simulink library "inp"  (Simulink 7.4)
settings: Solver=ode45  StartTime=0.0  StopTime=10.0  RelTol=1e-3
undefined symbols (not defined in the file): AINP_BrkPedalInterp_X_bar, C_TASK_10MS_S, ENUM_SHIFTER_D, ENUM_SHIFTER_N, ENUM_SHIFTER_P, ENUM_SHIFTER_R, KINP_BonnetCloseVehSpdThre_kph, KINP_EDUCoolantTempFilTm_s, KINP_EDUOilPressureFilTm_s, KINP_EDUOilTempFilTm_s, KINP_EDUSynchDisp_mm, KINP_EDUSynchPosnPWMDC_pct_LowerLimit, KINP_EDUSynchPosnPWMDC_pct_ovrdflg, KINP_EDUSynchPosnPWMDC_pct_ovrdval, KINP_EDUSynchPosnPWMDC_pct_UpperLimit, KINP_ShifterPosConfirmD_s, KINP_ShifterPosConfirmN_s, KINP_ShifterPosConfirmP_s, KINP_ShifterPosConfirmR_s, KINP_SingleAccPedalFltRateLim_pct, KINP_TMSpd2VehSpdSigNeg_rpm, KINP_TMSpd2VehSpdSigPos_rpm, KINP_ValidCheck_EDUSynchPosnPWMDC_dec, KINP_ValidCheck_EDUSynchPosnPWMDC_inc, KINP_ValidCheck_EDUSynchPosnPWMDC_lim, KINP_VehSpdSigKeepThres_kph, KPH2MPS, MIN2SEC, MINP_BrkPedalInterp_pct, MPS2KPH, PI, seat_version_control_block_callbacks, TIRE_RADIUS
libraries: inp_lib x166, hcu_lib x4, simulink x1
(part 3 of 9)

== system inp/INP/INP_100MS/Message (100ms) ISC_HSC2_FrP02 ==
  BHAL_IN_100ms : Inport
  BSRV_In_ovrdflgs : Inport  Port=2
  BSRV_In_ovrdvals : Inport  Port=3
  VINP_ISCMsgAlive_flg : Inport  Port=4
  Bus Creator : BusCreator  Inputs=6
  Bus Selector1 : BusSelector  OutputSignals=VSRV_ISGOverTempIn_flg_ovrdflg
  Bus Selector10 : BusSelector  OutputSignals=VHAL_ISGDeratingIn_flg
  Bus Selector12 : BusSelector  OutputSignals=VSRV_DCDCTempIn_C_ovrdflg
  Bus Selector14 : BusSelector  OutputSignals=VSRV_DCDCLVLoadIn_pct_ovrdflg
  Bus Selector16 : BusSelector  OutputSignals=VSRV_DCDCLVLoadIn_pct_ovrdval
  Bus Selector17 : BusSelector  OutputSignals=VHAL_DCDCLVLoadIn_pct
  Bus Selector2 : BusSelector  OutputSignals=VSRV_ISCHSC2FrP02Active_flg_ovrdflg
  Bus Selector3 : BusSelector  OutputSignals=VSRV_ISCHSC2FrP02Active_flg_ovrdval
  Bus Selector4 : BusSelector  OutputSignals=VHAL_DCDCTempValidIn_flg
  Bus Selector43 : BusSelector  OutputSignals=VSRV_DCDCFaultIn_flg_ovrdflg
  Bus Selector44 : BusSelector  OutputSignals=VSRV_DCDCFaultIn_flg_ovrdval
  Bus Selector45 : BusSelector  OutputSignals=VHAL_DCDCFaultIn_flg
  Bus Selector46 : BusSelector  OutputSignals=VSRV_DCDCTempIn_C_ovrdval
  Bus Selector47 : BusSelector  OutputSignals=VHAL_DCDCTempIn_C
  Bus Selector5 : BusSelector  OutputSignals=VSRV_ISGOverTempIn_flg_ovrdval
  Bus Selector6 : BusSelector  OutputSignals=VHAL_DCDCLVLoadValidIn_flg
  Bus Selector7 : BusSelector  OutputSignals=VHAL_ISGOverTempIn_flg
  Bus Selector8 : BusSelector  OutputSignals=VSRV_ISGDeratingIn_flg_ovrdflg
  Bus Selector9 : BusSelector  OutputSignals=VSRV_ISGDeratingIn_flg_ovrdval
  Subsys VINP_DCDCFault_flg : inp_lib/msgactv_ovrd  SystemSampleTime=-1  cal_ovrdflg=KINP_DCDCFault_flg_ovrdflg  cal_ovrdval=KINP_DCDCFault_flg_ovrdval  default=KINP_DCDCFaultDefault_flg
  Subsys VINP_DCDCLVLoad_pct : inp_lib/valid_msgactv_sat_ovrd  SystemSampleTime=-1  cal_ovrdflg=KINP_DCDCLVLoad_pct_ovrdflg  cal_ovrdval=KINP_DCDCLVLoad_pct_ovrdval  lim=KINP_ValidCheck_DCDCLVLoad_lim  inc=KINP_ValidCheck_DCDCLVLoad_inc  dec=KINP_ValidCheck_DCDCLVLoad_dec  default=KINP_DCDCLVLoadDefault_pct  hi=KINP_DCDCLVLoad_pct_Max  lo=KINP_DCDCLVLoad_pct_Min
  Subsys VINP_DCDCTemp_C : inp_lib/valid_msgactv_sat_ovrd  SystemSampleTime=-1  cal_ovrdflg=KINP_DCDCTemp_C_ovrdflg  cal_ovrdval=KINP_DCDCTemp_C_ovrdval  lim=KINP_ValidCheck_DCDCTemp_lim  inc=KINP_ValidCheck_DCDCTemp_inc  dec=KINP_ValidCheck_DCDCTemp_dec  default=KINP_DCDCTempDefault_C  hi=KINP_DCDCTemp_C_Max  lo=KINP_DCDCTemp_C_Min
  Subsys VINP_ISCHSC2FrP02Active_flg : inp_lib/override  SystemSampleTime=-1  cal_ovrdflg=KINP_ISCHSC2FrP02Active_ovrdflg  cal_ovrdval=KINP_ISCHSC2FrP02Active_flg_ovrdval
  Subsys VINP_ISGDerating_flg : inp_lib/msgactv_ovrd  SystemSampleTime=-1  cal_ovrdflg=KINP_ISGDerating_flg_ovrdflg  cal_ovrdval=KINP_ISGDerating_flg_ovrdval  default=KINP_ISGDeratingDefault_flg
  Subsys VINP_ISGOverTemp_flg : inp_lib/msgactv_ovrd  SystemSampleTime=-1  cal_ovrdflg=KINP_ISGOverTemp_flg_ovrdflg  cal_ovrdval=KINP_ISGOverTemp_flg_ovrdval  default=KINP_ISGOverTempDefault_flg
  Terminator{,1..4} (5 alike) : Terminator
  BINP_ISC_HSC2_FrP02 : Outport
  wires:
  [BSRV_In_ovrdvals] -> Bus Selector9/1
  [BSRV_In_ovrdflgs] -> Bus Selector8/1
  [BSRV_In_ovrdvals] -> Bus Selector5/1
  [BSRV_In_ovrdflgs] -> Bus Selector1/1
  [BSRV_In_ovrdvals] -> Bus Selector3/1
  [BSRV_In_ovrdflgs] -> Bus Selector2/1
  [BSRV_In_ovrdvals] -> Bus Selector46/1
  [BSRV_In_ovrdflgs] -> Bus Selector12/1
  [BSRV_In_ovrdvals] -> Bus Selector44/1
  [BSRV_In_ovrdflgs] -> Bus Selector43/1
  BHAL_IN_100ms/1 -> Bus Selector10/1, Bus Selector7/1, Bus Selector47/1, Bus Selector4/1, Bus Selector6/1, Bus Selector17/1, Bus Selector45/1
  Bus Creator/1 -> BINP_ISC_HSC2_FrP02/1  "BINP_ISC_HSC2_FrP02"
  BSRV_In_ovrdvals/1 -> [BSRV_In_ovrdvals]
  BSRV_In_ovrdflgs/1 -> [BSRV_In_ovrdflgs]
  VINP_ISCMsgAlive_flg/1 -> [VINP_ISCMsgAlive_flg]
  [BSRV_In_ovrdvals] -> Bus Selector16/1
  [BSRV_In_ovrdflgs] -> Bus Selector14/1
  Bus Selector45/1 -> Subsys VINP_DCDCFault_flg/1  "<VHAL_DCDCFaultIn_flg>"
  Bus Selector43/1 -> Subsys VINP_DCDCFault_flg/2  "<VSRV_DCDCFaultIn_flg_ovrdflg>"
  Bus Selector44/1 -> Subsys VINP_DCDCFault_flg/3  "<VSRV_DCDCFaultIn_flg_ovrdval>"
  [MsgAlive_flgs] -> Subsys VINP_DCDCFault_flg/4
  Subsys VINP_DCDCFault_flg/1 -> Bus Creator/3  "VINP_DCDCFault_flg"
  Subsys VINP_DCDCFault_flg/2 -> Terminator/1
  Bus Selector17/1 -> Subsys VINP_DCDCLVLoad_pct/1  "<VHAL_DCDCLVLoadIn_pct>"
  Bus Selector6/1 -> Subsys VINP_DCDCLVLoad_pct/2  "<VHAL_DCDCLVLoadValidIn_flg>"
  Bus Selector14/1 -> Subsys VINP_DCDCLVLoad_pct/3  "<VSRV_DCDCLVLoadIn_pct_ovrdflg>"
  Bus Selector16/1 -> Subsys VINP_DCDCLVLoad_pct/4  "<VSRV_DCDCLVLoadIn_pct_ovrdval>"
  [MsgAlive_flgs] -> Subsys VINP_DCDCLVLoad_pct/5
  Subsys VINP_DCDCLVLoad_pct/1 -> Bus Creator/5  "VINP_DCDCLVLoad_pct"
  Subsys VINP_DCDCLVLoad_pct/2 -> Terminator1/1
  Bus Selector47/1 -> Subsys VINP_DCDCTemp_C/1  "<VHAL_DCDCTempIn_C>"
  Bus Selector4/1 -> Subsys VINP_DCDCTemp_C/2  "<VHAL_DCDCTempValidIn_flg>"
  Bus Selector12/1 -> Subsys VINP_DCDCTemp_C/3  "<VSRV_DCDCTempIn_C_ovrdflg>"
  Bus Selector46/1 -> Subsys VINP_DCDCTemp_C/4  "<VSRV_DCDCTempIn_C_ovrdval>"
  [MsgAlive_flgs] -> Subsys VINP_DCDCTemp_C/5
  Subsys VINP_DCDCTemp_C/1 -> Bus Creator/4  "VINP_DCDCTemp_C"
  Subsys VINP_DCDCTemp_C/2 -> Terminator2/1
  Bus Selector2/1 -> Subsys VINP_ISCHSC2FrP02Active_flg/2  "<VSRV_ISCHSC2FrP02Active_flg_ovrdflg>"
  Bus Selector3/1 -> Subsys VINP_ISCHSC2FrP02Active_flg/3  "<VSRV_ISCHSC2FrP02Active_flg_ovrdval>"
  Subsys VINP_ISCHSC2FrP02Active_flg/1 -> Bus Creator/6  "VINP_ISCHSC2FrP02Active_flg"
  Bus Selector10/1 -> Subsys VINP_ISGDerating_flg/1  "<VHAL_ISGDeratingIn_flg>"
  Bus Selector8/1 -> Subsys VINP_ISGDerating_flg/2  "<VSRV_ISGDeratingIn_flg_ovrdflg>"
  Bus Selector9/1 -> Subsys VINP_ISGDerating_flg/3  "<VSRV_ISGDeratingIn_flg_ovrdval>"
  [MsgAlive_flgs] -> Subsys VINP_ISGDerating_flg/4  "MsgAlive_flgs"
  Subsys VINP_ISGDerating_flg/1 -> Bus Creator/1  "VINP_ISGDerating_flg"
  Subsys VINP_ISGDerating_flg/2 -> Terminator3/1
  Bus Selector7/1 -> Subsys VINP_ISGOverTemp_flg/1  "<VHAL_ISGOverTempIn_flg>"
  Bus Selector1/1 -> Subsys VINP_ISGOverTemp_flg/2  "<VSRV_ISGOverTempIn_flg_ovrdflg>"
  Bus Selector5/1 -> Subsys VINP_ISGOverTemp_flg/3  "<VSRV_ISGOverTempIn_flg_ovrdval>"
  [MsgAlive_flgs] -> Subsys VINP_ISGOverTemp_flg/4  "MsgAlive_flgs"
  Subsys VINP_ISGOverTemp_flg/1 -> Bus Creator/2  "VINP_ISGOverTemp_flg"
  Subsys VINP_ISGOverTemp_flg/2 -> Terminator4/1
  [VINP_ISCMsgAlive_flg] -> Subsys VINP_ISCHSC2FrP02Active_flg/1, [MsgAlive_flgs]  "VINP_ISCMsgAlive_flg"

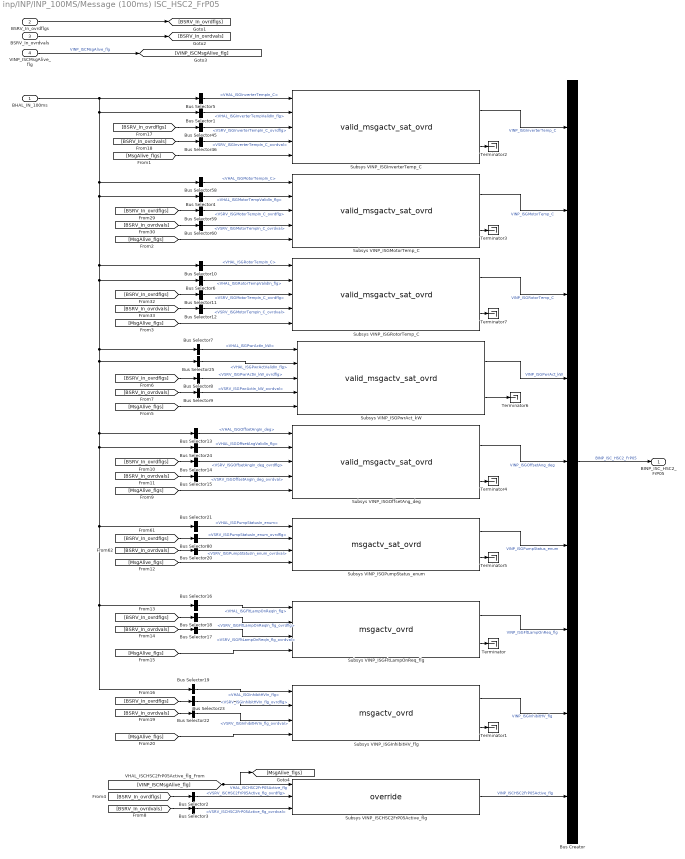
== system inp/INP/INP_100MS/Message (100ms) ISC_HSC2_FrP05 ==
  BHAL_IN_100ms : Inport
  BSRV_In_ovrdflgs : Inport  Port=2
  BSRV_In_ovrdvals : Inport  Port=3
  VINP_ISCMsgAlive_flg : Inport  Port=4
  Bus Creator : BusCreator  Inputs=9
  Bus Selector1 : BusSelector  OutputSignals=VHAL_ISGInverterTempValidIn_flg
  Bus Selector10 : BusSelector  OutputSignals=VHAL_ISGRotorTempIn_C
  Bus Selector11 : BusSelector  OutputSignals=VSRV_ISGMotorTempIn_C_ovrdflg
  Bus Selector12 : BusSelector  OutputSignals=VSRV_ISGMotorTempIn_C_ovrdval
  Bus Selector13 : BusSelector  OutputSignals=VHAL_ISGOffsetAngIn_deg
  Bus Selector14 : BusSelector  OutputSignals=VSRV_ISGOffsetAngIn_deg_ovrdflg
  Bus Selector15 : BusSelector  OutputSignals=VSRV_ISGOffsetAngIn_deg_ovrdval
  Bus Selector16 : BusSelector  OutputSignals=VHAL_ISGFltLampOnReqIn_flg
  Bus Selector17 : BusSelector  OutputSignals=VSRV_ISGFltLampOnReqIn_flg_ovrdval
  Bus Selector18 : BusSelector  OutputSignals=VSRV_ISGFltLampOnReqIn_flg_ovrdflg
  Bus Selector19 : BusSelector  OutputSignals=VHAL_ISGInhibitHVIn_flg
  Bus Selector2 : BusSelector  OutputSignals=VSRV_ISCHSC2FrP05Active_flg_ovrdflg
  Bus Selector20 : BusSelector  OutputSignals=VSRV_ISGPumpStatusIn_enum_ovrdval
  Bus Selector21 : BusSelector  OutputSignals=VHAL_ISGPumpStatusIn_enum
  Bus Selector22 : BusSelector  OutputSignals=VSRV_ISGInhibitHVIn_flg_ovrdval
  Bus Selector23 : BusSelector  OutputSignals=VSRV_ISGInhibitHVIn_flg_ovrdflg
  Bus Selector24 : BusSelector  OutputSignals=VHAL_ISGOffsetAngValidIn_flg
  Bus Selector25 : BusSelector  OutputSignals=VHAL_ISGPwrActValidIn_flg
  Bus Selector3 : BusSelector  OutputSignals=VSRV_ISCHSC2FrP05Active_flg_ovrdval
  Bus Selector4 : BusSelector  OutputSignals=VHAL_ISGMotorTempValidIn_flg
  Bus Selector45 : BusSelector  OutputSignals=VSRV_ISGInverterTempIn_C_ovrdflg
  Bus Selector46 : BusSelector  OutputSignals=VSRV_ISGInverterTempIn_C_ovrdval
  Bus Selector5 : BusSelector  OutputSignals=VHAL_ISGInverterTempIn_C
  Bus Selector58 : BusSelector  OutputSignals=VHAL_ISGMotorTempIn_C
  Bus Selector59 : BusSelector  OutputSignals=VSRV_ISGMotorTempIn_C_ovrdflg
  Bus Selector6 : BusSelector  OutputSignals=VHAL_ISGRotorTempValidIn_flg
  Bus Selector60 : BusSelector  OutputSignals=VSRV_ISGMotorTempIn_C_ovrdval
  Bus Selector7 : BusSelector  OutputSignals=VHAL_ISGPwrActIn_kW
  Bus Selector8 : BusSelector  OutputSignals=VSRV_ISGPwrActIn_kW_ovrdflg
  Bus Selector80 : BusSelector  OutputSignals=VSRV_ISGPumpStatusIn_enum_ovrdflg
  Bus Selector9 : BusSelector  OutputSignals=VSRV_ISGPwrActIn_kW_ovrdval
  Subsys VINP_ISCHSC2FrP05Active_flg : inp_lib/override  SystemSampleTime=-1  cal_ovrdflg=KINP_ISCHSC2FrP05Active_ovrdflg  cal_ovrdval=KINP_ISCHSC2FrP05Active_flg_ovrdval
  Subsys VINP_ISGFltLampOnReq_flg : inp_lib/msgactv_ovrd  SystemSampleTime=-1  cal_ovrdflg=KINP_ISGFltLampOnReq_flg_ovrdflg  cal_ovrdval=KINP_ISGFltLampOnReq_flg_ovrdval  default=KINP_ISGFltLampOnReqDefault_flg
  Subsys VINP_ISGInhibitHV_flg : inp_lib/msgactv_ovrd  SystemSampleTime=-1  cal_ovrdflg=KINP_ISGInhibitHV_flg_ovrdflg  cal_ovrdval=KINP_ISGInhibitHV_flg_ovrdval  default=KINP_ISGInhibitHVDefault_flg
  Subsys VINP_ISGInverterTemp_C : inp_lib/valid_msgactv_sat_ovrd  SystemSampleTime=-1  cal_ovrdflg=KINP_ISGInverterTemp_C_ovrdflg  cal_ovrdval=KINP_ISGInverterTemp_C_ovrdval  lim=KINP_ValidCheck_ISGInverterTemp_lim  inc=KINP_ValidCheck_ISGInverterTemp_inc  dec=KINP_ValidCheck_ISGInverterTemp_dec  default=KINP_ISGInverterTempDefault_C  hi=KINP_ISGInverterTemp_C_Max  lo=KINP_ISGInverterTemp_C_Min
  Subsys VINP_ISGMotorTemp_C : inp_lib/valid_msgactv_sat_ovrd  SystemSampleTime=-1  cal_ovrdflg=KINP_ISGMotorTemp_C_ovrdflg  cal_ovrdval=KINP_ISGMotorTemp_C_ovrdval  lim=KINP_ValidCheck_ISGMotorTemp_lim  inc=KINP_ValidCheck_ISGMotorTemp_inc  dec=KINP_ValidCheck_ISGMotorTemp_dec  default=KINP_ISGMotorTempDefault_C  hi=KINP_ISGMotorTemp_C_Max  lo=KINP_ISGMotorTemp_C_Min
  Subsys VINP_ISGOffsetAng_deg : inp_lib/valid_msgactv_sat_ovrd  SystemSampleTime=-1  cal_ovrdflg=KINP_ISGOffsetAng_deg_ovrdflg  cal_ovrdval=KINP_ISGOffsetAng_deg_ovrdval  lim=KINP_ValidCheck_ISGOffsetAng_lim  inc=KINP_ValidCheck_ISGOffsetAng_inc  dec=KINP_ValidCheck_ISGOffsetAng_dec  default=KINP_ISGOffsetAngDefault_deg  hi=KINP_ISGOffsetAng_deg_Max  lo=KINP_ISGOffsetAng_deg_Min
  Subsys VINP_ISGPumpStatus_enum : inp_lib/msgactv_sat_ovrd  SystemSampleTime=-1  cal_ovrdflg=KINP_ISGPumpStatus_enum_ovrdflg  cal_ovrdval=KINP_ISGPumpStatus_enum_ovrdval  default=KINP_ISGPumpStatusDefault_enum  hi=KINP_ISGPumpStatus_enum_Max  lo=KINP_ISGPumpStatus_enum_Min
  Subsys VINP_ISGPwrAct_kW : inp_lib/valid_msgactv_sat_ovrd  SystemSampleTime=-1  cal_ovrdflg=KINP_ISGPwrAct_kW_ovrdflg  cal_ovrdval=KINP_ISGPwrAct_kW_ovrdval  lim=KINP_ValidCheck_ISGPwrAct_lim  inc=KINP_ValidCheck_ISGPwrAct_inc  dec=KINP_ValidCheck_ISGPwrAct_dec  default=KINP_ISGPwrActDefault_kW  hi=KINP_ISGPwrAct_kW_Max  lo=KINP_ISGPwrAct_kW_Min
  Subsys VINP_ISGRotorTemp_C : inp_lib/valid_msgactv_sat_ovrd  SystemSampleTime=-1  cal_ovrdflg=KINP_ISGRotorTemp_C_ovrdflg  cal_ovrdval=KINP_ISGRotorTemp_C_ovrdval  lim=KINP_ValidCheck_ISGRotorTemp_lim  inc=KINP_ValidCheck_ISGRotorTemp_inc  dec=KINP_ValidCheck_ISGRotorTemp_dec  default=KINP_ISGRotorTempDefault_C  hi=KINP_ISGRotorTemp_C_Max  lo=KINP_ISGRotorTemp_C_Min
  Terminator{,1..7} (8 alike) : Terminator
  BINP_ISC_HSC2_FrP05 : Outport
  wires:
  Bus Selector24/1 -> Subsys VINP_ISGOffsetAng_deg/2  "<VHAL_ISGOffsetAngValidIn_flg>"
  Bus Selector25/1 -> Subsys VINP_ISGPwrAct_kW/2  "<VHAL_ISGPwrActValidIn_flg>"
  Bus Selector14/1 -> Subsys VINP_ISGOffsetAng_deg/3  "<VSRV_ISGOffsetAngIn_deg_ovrdflg>"
  [BSRV_In_ovrdvals] -> Bus Selector22/1
  [BSRV_In_ovrdflgs] -> Bus Selector23/1
  [BSRV_In_ovrdvals] -> Bus Selector17/1
  [BSRV_In_ovrdflgs] -> Bus Selector18/1
  [BSRV_In_ovrdvals] -> Bus Selector3/1
  [BSRV_In_ovrdflgs] -> Bus Selector2/1
  [VINP_ISCMsgAlive_flg] -> [MsgAlive_flgs], Subsys VINP_ISCHSC2FrP05Active_flg/1  "VHAL_ISCHSC2FrP05Active_flg"
  [BSRV_In_ovrdflgs] -> Bus Selector80/1
  [BSRV_In_ovrdvals] -> Bus Selector20/1
  BHAL_IN_100ms/1 -> Bus Selector1/1, Bus Selector10/1, Bus Selector6/1, Bus Selector25/1, Bus Selector24/1, Bus Selector19/1, Bus Selector16/1, Bus Selector21/1, Bus Selector13/1, Bus Selector7/1, Bus Selector4/1, Bus Selector58/1, Bus Selector5/1
  [BSRV_In_ovrdvals] -> Bus Selector12/1
  [BSRV_In_ovrdflgs] -> Bus Selector11/1
  [BSRV_In_ovrdvals] -> Bus Selector60/1
  [BSRV_In_ovrdflgs] -> Bus Selector59/1
  [BSRV_In_ovrdvals] -> Bus Selector46/1
  [BSRV_In_ovrdflgs] -> Bus Selector45/1
  VINP_ISCMsgAlive_flg/1 -> [VINP_ISCMsgAlive_flg]  "VINP_ISCMsgAlive_flg"
  BSRV_In_ovrdflgs/1 -> [BSRV_In_ovrdflgs]
  BSRV_In_ovrdvals/1 -> [BSRV_In_ovrdvals]
  Bus Creator/1 -> BINP_ISC_HSC2_FrP05/1  "BINP_ISC_HSC2_FrP05"
  [BSRV_In_ovrdvals] -> Bus Selector9/1
  [BSRV_In_ovrdflgs] -> Bus Selector8/1
  [BSRV_In_ovrdvals] -> Bus Selector15/1
  [BSRV_In_ovrdflgs] -> Bus Selector14/1
  Bus Selector2/1 -> Subsys VINP_ISCHSC2FrP05Active_flg/2  "<VSRV_ISCHSC2FrP05Active_flg_ovrdflg>"
  Bus Selector3/1 -> Subsys VINP_ISCHSC2FrP05Active_flg/3  "<VSRV_ISCHSC2FrP05Active_flg_ovrdval>"
  Subsys VINP_ISCHSC2FrP05Active_flg/1 -> Bus Creator/9  "VINP_ISCHSC2FrP05Active_flg"
  Bus Selector16/1 -> Subsys VINP_ISGFltLampOnReq_flg/1  "<VHAL_ISGFltLampOnReqIn_flg>"
  Bus Selector18/1 -> Subsys VINP_ISGFltLampOnReq_flg/2  "<VSRV_ISGFltLampOnReqIn_flg_ovrdflg>"
  Bus Selector17/1 -> Subsys VINP_ISGFltLampOnReq_flg/3  "<VSRV_ISGFltLampOnReqIn_flg_ovrdval>"
  [MsgAlive_flgs] -> Subsys VINP_ISGFltLampOnReq_flg/4
  Subsys VINP_ISGFltLampOnReq_flg/1 -> Bus Creator/7  "VINP_ISGFltLampOnReq_flg"
  Subsys VINP_ISGFltLampOnReq_flg/2 -> Terminator/1
  Bus Selector19/1 -> Subsys VINP_ISGInhibitHV_flg/1  "<VHAL_ISGInhibitHVIn_flg>"
  Bus Selector23/1 -> Subsys VINP_ISGInhibitHV_flg/2  "<VSRV_ISGInhibitHVIn_flg_ovrdflg>"
  Bus Selector22/1 -> Subsys VINP_ISGInhibitHV_flg/3  "<VSRV_ISGInhibitHVIn_flg_ovrdval>"
  [MsgAlive_flgs] -> Subsys VINP_ISGInhibitHV_flg/4
  Subsys VINP_ISGInhibitHV_flg/1 -> Bus Creator/8  "VINP_ISGInhibitHV_flg"
  Subsys VINP_ISGInhibitHV_flg/2 -> Terminator1/1
  Bus Selector5/1 -> Subsys VINP_ISGInverterTemp_C/1  "<VHAL_ISGInverterTempIn_C>"
  Bus Selector1/1 -> Subsys VINP_ISGInverterTemp_C/2  "<VHAL_ISGInverterTempValidIn_flg>"
  Bus Selector45/1 -> Subsys VINP_ISGInverterTemp_C/3  "<VSRV_ISGInverterTempIn_C_ovrdflg>"
  Bus Selector46/1 -> Subsys VINP_ISGInverterTemp_C/4  "<VSRV_ISGInverterTempIn_C_ovrdval>"
  [MsgAlive_flgs] -> Subsys VINP_ISGInverterTemp_C/5
  Subsys VINP_ISGInverterTemp_C/1 -> Bus Creator/1  "VINP_ISGInverterTemp_C"
  Subsys VINP_ISGInverterTemp_C/2 -> Terminator2/1
  Bus Selector58/1 -> Subsys VINP_ISGMotorTemp_C/1  "<VHAL_ISGMotorTempIn_C>"
  Bus Selector4/1 -> Subsys VINP_ISGMotorTemp_C/2  "<VHAL_ISGMotorTempValidIn_flg>"
  Bus Selector59/1 -> Subsys VINP_ISGMotorTemp_C/3  "<VSRV_ISGMotorTempIn_C_ovrdflg>"
  Bus Selector60/1 -> Subsys VINP_ISGMotorTemp_C/4  "<VSRV_ISGMotorTempIn_C_ovrdval>"
  [MsgAlive_flgs] -> Subsys VINP_ISGMotorTemp_C/5
  Subsys VINP_ISGMotorTemp_C/1 -> Bus Creator/2  "VINP_ISGMotorTemp_C"
  Subsys VINP_ISGMotorTemp_C/2 -> Terminator3/1
  Bus Selector13/1 -> Subsys VINP_ISGOffsetAng_deg/1  "<VHAL_ISGOffsetAngIn_deg>"
  Bus Selector15/1 -> Subsys VINP_ISGOffsetAng_deg/4  "<VSRV_ISGOffsetAngIn_deg_ovrdval>"
  [MsgAlive_flgs] -> Subsys VINP_ISGOffsetAng_deg/5
  Subsys VINP_ISGOffsetAng_deg/1 -> Bus Creator/5  "VINP_ISGOffsetAng_deg"
  Subsys VINP_ISGOffsetAng_deg/2 -> Terminator4/1
  Bus Selector21/1 -> Subsys VINP_ISGPumpStatus_enum/1  "<VHAL_ISGPumpStatusIn_enum>"
  Bus Selector80/1 -> Subsys VINP_ISGPumpStatus_enum/2  "<VSRV_ISGPumpStatusIn_enum_ovrdflg>"
  Bus Selector20/1 -> Subsys VINP_ISGPumpStatus_enum/3  "<VSRV_ISGPumpStatusIn_enum_ovrdval>"
  [MsgAlive_flgs] -> Subsys VINP_ISGPumpStatus_enum/4
  Subsys VINP_ISGPumpStatus_enum/1 -> Bus Creator/6  "VINP_ISGPumpStatus_enum"
  Subsys VINP_ISGPumpStatus_enum/2 -> Terminator5/1
  Bus Selector7/1 -> Subsys VINP_ISGPwrAct_kW/1  "<VHAL_ISGPwrActIn_kW>"
  Bus Selector8/1 -> Subsys VINP_ISGPwrAct_kW/3  "<VSRV_ISGPwrActIn_kW_ovrdflg>"
  Bus Selector9/1 -> Subsys VINP_ISGPwrAct_kW/4  "<VSRV_ISGPwrActIn_kW_ovrdval>"
  [MsgAlive_flgs] -> Subsys VINP_ISGPwrAct_kW/5
  Subsys VINP_ISGPwrAct_kW/1 -> Bus Creator/4  "VINP_ISGPwrAct_kW"
  Subsys VINP_ISGPwrAct_kW/2 -> Terminator6/1
  Bus Selector10/1 -> Subsys VINP_ISGRotorTemp_C/1  "<VHAL_ISGRotorTempIn_C>"
  Bus Selector6/1 -> Subsys VINP_ISGRotorTemp_C/2  "<VHAL_ISGRotorTempValidIn_flg>"
  Bus Selector11/1 -> Subsys VINP_ISGRotorTemp_C/3  "<VSRV_ISGMotorTempIn_C_ovrdflg>"
  Bus Selector12/1 -> Subsys VINP_ISGRotorTemp_C/4  "<VSRV_ISGMotorTempIn_C_ovrdval>"
  [MsgAlive_flgs] -> Subsys VINP_ISGRotorTemp_C/5
  Subsys VINP_ISGRotorTemp_C/1 -> Bus Creator/3  "VINP_ISGRotorTemp_C"
  Subsys VINP_ISGRotorTemp_C/2 -> Terminator7/1

== system inp/INP/INP_100MS/Message (100ms) PMU_HSC_FrP00 ==
  BHAL_IN_100ms : Inport
  BSRV_In_ovrdflgs : Inport  Port=2
  BSRV_In_ovrdvals : Inport  Port=3
  VINP_PMUMsgAlive_flg : Inport  Port=4
  Bus Creator : BusCreator  Inputs=2
  Bus Selector1 : BusSelector  OutputSignals=VHAL_DCDCVoltSetptValidIn_flg
  Bus Selector10 : BusSelector  OutputSignals=VSRV_DCDCVoltSetptIn_V_ovrdval
  Bus Selector2 : BusSelector  OutputSignals=VSRV_PMUHSCFrP00Active_flg_ovrdflg
  Bus Selector3 : BusSelector  OutputSignals=VSRV_PMUHSCFrP00Active_flg_ovrdval
  Bus Selector7 : BusSelector  OutputSignals=VHAL_DCDCVoltSetptIn_V
  Bus Selector9 : BusSelector  OutputSignals=VSRV_DCDCVoltSetptIn_V_ovrdflg
  Subsys VINP_DCDCVoltSetpt_V : inp_lib/valid_msgactv_sat_ovrd  SystemSampleTime=-1  cal_ovrdflg=KINP_DCDCVoltSetpt_V_ovrdflg  cal_ovrdval=KINP_DCDCVoltSetpt_V_ovrdval  lim=KINP_ValidCheck_DCDCVoltSetpt_lim  inc=KINP_ValidCheck_DCDCVoltSetpt_inc  dec=KINP_ValidCheck_DCDCVoltSetpt_dec  default=KINP_DCDCVoltSetptDefault_V  hi=KINP_DCDCVoltSetpt_V_Max  lo=KINP_DCDCVoltSetpt_V_Min
  Subsys VINP_PMUHSCFrP00Active_flg : inp_lib/override  SystemSampleTime=-1  cal_ovrdflg=KINP_PMUHSCFrP00Active_ovrdflg  cal_ovrdval=KINP_PMUHSCFrP00Active_flg_ovrdval
  Terminator : Terminator
  BINP_PMU_HSC_FrP00 : Outport
  wires:
  [BSRV_In_ovrdvals] -> Bus Selector3/1
  [BSRV_In_ovrdflgs] -> Bus Selector2/1
  [VINP_PMUMsgAlive_flg] -> [MsgAlive_flgs], Subsys VINP_PMUHSCFrP00Active_flg/1  "VINP_PMUMsgAlive_flg"
  [BSRV_In_ovrdvals] -> Bus Selector10/1
  [BSRV_In_ovrdflgs] -> Bus Selector9/1
  BHAL_IN_100ms/1 -> Bus Selector1/1, Bus Selector7/1
  Bus Creator/1 -> BINP_PMU_HSC_FrP00/1  "BINP_PMU_HSC_FrP00"
  BSRV_In_ovrdvals/1 -> [BSRV_In_ovrdvals]
  BSRV_In_ovrdflgs/1 -> [BSRV_In_ovrdflgs]
  VINP_PMUMsgAlive_flg/1 -> [VINP_PMUMsgAlive_flg]  "VINP_PMUMsgAlive_flg"
  Bus Selector7/1 -> Subsys VINP_DCDCVoltSetpt_V/1  "<VHAL_DCDCVoltSetptIn_V>"
  Bus Selector1/1 -> Subsys VINP_DCDCVoltSetpt_V/2  "<VHAL_DCDCVoltSetptValidIn_flg>"
  Bus Selector9/1 -> Subsys VINP_DCDCVoltSetpt_V/3  "<VSRV_DCDCVoltSetptIn_V_ovrdflg>"
  Bus Selector10/1 -> Subsys VINP_DCDCVoltSetpt_V/4  "<VSRV_DCDCVoltSetptIn_V_ovrdval>"
  [MsgAlive_flgs] -> Subsys VINP_DCDCVoltSetpt_V/5
  Subsys VINP_DCDCVoltSetpt_V/1 -> Bus Creator/1  "VINP_DCDCVoltSetpt_V"
  Subsys VINP_DCDCVoltSetpt_V/2 -> Terminator/1
  Bus Selector2/1 -> Subsys VINP_PMUHSCFrP00Active_flg/2  "<VSRV_PMUHSCFrP00Active_flg_ovrdflg>"
  Bus Selector3/1 -> Subsys VINP_PMUHSCFrP00Active_flg/3  "<VSRV_PMUHSCFrP00Active_flg_ovrdval>"
  Subsys VINP_PMUHSCFrP00Active_flg/1 -> Bus Creator/2  "VINP_PMUHSCFrP00Active_flg"

== system inp/INP/INP_100MS/Message (100ms) SMU_HSC_FrP06 ==
  BHAL_IN_100ms : Inport
  BSRV_In_ovrdflgs : Inport  Port=2
  BSRV_In_ovrdvals : Inport  Port=3
  VINP_SMUMsgAlive_flg : Inport  Port=4
  Bus Creator : BusCreator  Inputs=6
  Bus Selector1 : BusSelector  OutputSignals=VSRV_SMUHSCFrP06Active_flg_ovrdflg
  Bus Selector10 : BusSelector  OutputSignals=VHAL_ACCompressorPowerValidIn_flg
  Bus Selector13 : BusSelector  OutputSignals=VSRV_ATCEngOnReqIn_enum_ovrdflg
  Bus Selector14 : BusSelector  OutputSignals=VSRV_ATCEngOnReqIn_enum_ovrdval
  Bus Selector17 : BusSelector  OutputSignals=VHAL_ATCEngOnReqIn_enum
  Bus Selector2 : BusSelector  OutputSignals=VHAL_BonnetOpenIn_flg
  Bus Selector20 : BusSelector  OutputSignals=VSRV_ACCompressorPowerIn_kW_ovrdflg
  Bus Selector23 : BusSelector  OutputSignals=VSRV_ACCompressorPowerIn_kW_ovrdval
  Bus Selector3 : BusSelector  OutputSignals=VSRV_SMUHSCFrP06Active_flg_ovrdval
  Bus Selector4 : BusSelector  OutputSignals=VHAL_DriverDoorOpenIn_flg
  Bus Selector5 : BusSelector  OutputSignals=VSRV_BonnetOpenIn_flg_ovrdval
  Bus Selector6 : BusSelector  OutputSignals=VHAL_ACCompressorPowerIn_kW
  Bus Selector7 : BusSelector  OutputSignals=VSRV_DriverDoorOpenIn_flg_ovrdval
  Bus Selector8 : BusSelector  OutputSignals=VSRV_BonnetOpenIn_flg_ovrdflg
  Bus Selector9 : BusSelector  OutputSignals=VSRV_DriverDoorOpenIn_flg_ovrdflg
  Subsys VINP_ATCEngOnReq_enum : inp_lib/msgactv_sat_ovrd  SystemSampleTime=-1  cal_ovrdflg=KINP_ATCEngOnReq_enum_ovrdflg  cal_ovrdval=KINP_ATCEngOnReq_enum_ovrdval  default=KINP_ATCEngOnReqDefault_enum  hi=KINP_ATCEngOnReq_enum_Max  lo=KINP_ATCEngOnReq_enum_Min
  Subsys VINP_BonnetOpen_flg : inp_lib/msgactv_ovrd  SystemSampleTime=-1  cal_ovrdflg=KINP_BonnetOpen_flg_ovrdflg  cal_ovrdval=KINP_BonnetOpen_flg_ovrdval  default=KINP_BonnetOpenDefault_flg
  Subsys VINP_DriverDoorOpen_flg : inp_lib/msgactv_ovrd  SystemSampleTime=-1  cal_ovrdflg=KINP_DriverDoorOpen_flg_ovrdflg  cal_ovrdval=KINP_DriverDoorOpen_flg_ovrdval  default=KINP_DriverDoorOpenDefault_flg
  Subsys VINP_HVBattEnergyAvail_kWh : inp_lib/valid_msgactv_sat_ovrd  SystemSampleTime=-1  cal_ovrdflg=KINP_ACCompressorPower_kW_ovrdflg  cal_ovrdval=KINP_ACCompressorPower_kW_ovrdval  lim=KINP_ValidCheck_ACCompressorPower_lim  inc=KINP_ValidCheck_ACCompressorPower_inc  dec=KINP_ValidCheck_ACCompressorPower_dec  default=KINP_ACCompressorPowerDefault_kW  hi=KINP_ACCompressorPower_kW_Max  lo=KINP_ACCompressorPower_kW_Min
  Subsys VINP_SMUHSCFrP06Active_flg : inp_lib/override  SystemSampleTime=-1  cal_ovrdflg=KINP_SMUHSCFrP06Active_ovrdflg  cal_ovrdval=KINP_SMUHSCFrP06Active_flg_ovrdval
  Terminator : Terminator
  Terminator1 : Terminator
  Terminator2 : Terminator
  BINP_SMU_HSC_FrP06 : Outport
  wires:
  Bus Selector10/1 -> Subsys VINP_HVBattEnergyAvail_kWh/2  "<VHAL_ACCompressorPowerValidIn_flg>"
  [BSRV_In_ovrdvals] -> Bus Selector3/1
  [BSRV_In_ovrdflgs] -> Bus Selector1/1
  [VINP_SMUMsgAlive_flg] -> [MsgAlive_flgs], Subsys VINP_SMUHSCFrP06Active_flg/1
  [BSRV_In_ovrdflgs] -> Bus Selector13/1
  [BSRV_In_ovrdvals] -> Bus Selector14/1
  BHAL_IN_100ms/1 -> Bus Selector10/1, Bus Selector6/1, Bus Selector17/1, Bus Selector2/1, Bus Selector4/1
  [BSRV_In_ovrdvals] -> Bus Selector7/1
  [BSRV_In_ovrdflgs] -> Bus Selector9/1
  [BSRV_In_ovrdvals] -> Bus Selector5/1
  [BSRV_In_ovrdflgs] -> Bus Selector8/1
  Bus Creator/1 -> BINP_SMU_HSC_FrP06/1  "BINP_SMU_HSC_FrP06"
  BSRV_In_ovrdvals/1 -> [BSRV_In_ovrdvals]
  BSRV_In_ovrdflgs/1 -> [BSRV_In_ovrdflgs]
  VINP_SMUMsgAlive_flg/1 -> [VINP_SMUMsgAlive_flg]
  [BSRV_In_ovrdflgs] -> Bus Selector20/1
  [BSRV_In_ovrdvals] -> Bus Selector23/1
  Bus Selector6/1 -> Subsys VINP_HVBattEnergyAvail_kWh/1  "<VHAL_ACCompressorPowerIn_kW>"
  Bus Selector20/1 -> Subsys VINP_HVBattEnergyAvail_kWh/3  "<VSRV_ACCompressorPowerIn_kW_ovrdflg>"
  Bus Selector23/1 -> Subsys VINP_HVBattEnergyAvail_kWh/4  "<VSRV_ACCompressorPowerIn_kW_ovrdval>"
  [MsgAlive_flgs] -> Subsys VINP_HVBattEnergyAvail_kWh/5
  Subsys VINP_HVBattEnergyAvail_kWh/1 -> Bus Creator/5  "VINP_ACCompressorPower_kW"
  Subsys VINP_HVBattEnergyAvail_kWh/2 -> Terminator/1
  Bus Selector17/1 -> Subsys VINP_ATCEngOnReq_enum/1  "<VHAL_ATCEngOnReqIn_enum>"
  Bus Selector13/1 -> Subsys VINP_ATCEngOnReq_enum/2  "<VSRV_ATCEngOnReqIn_enum_ovrdflg>"
  Bus Selector14/1 -> Subsys VINP_ATCEngOnReq_enum/3  "<VSRV_ATCEngOnReqIn_enum_ovrdval>"
  [MsgAlive_flgs] -> Subsys VINP_ATCEngOnReq_enum/4
  Subsys VINP_ATCEngOnReq_enum/1 -> Bus Creator/4  "VINP_ATCEngOnReq_enum"
  Subsys VINP_ATCEngOnReq_enum/2 -> Terminator1/1
  Bus Selector4/1 -> Subsys VINP_DriverDoorOpen_flg/1  "<VHAL_DriverDoorOpenIn_flg>"
  Bus Selector9/1 -> Subsys VINP_DriverDoorOpen_flg/2  "<VSRV_DriverDoorOpenIn_flg_ovrdflg>"
  Bus Selector7/1 -> Subsys VINP_DriverDoorOpen_flg/3  "<VSRV_DriverDoorOpenIn_flg_ovrdval>"
  [MsgAlive_flgs] -> Subsys VINP_DriverDoorOpen_flg/4
  Subsys VINP_DriverDoorOpen_flg/1 -> Bus Creator/1  "VINP_DriverDoorOpen_flg"
  Subsys VINP_DriverDoorOpen_flg/2 -> Terminator2/1
  Bus Selector1/1 -> Subsys VINP_SMUHSCFrP06Active_flg/2  "<VSRV_SMUHSCFrP06Active_flg_ovrdflg>"
  Bus Selector3/1 -> Subsys VINP_SMUHSCFrP06Active_flg/3  "<VSRV_SMUHSCFrP06Active_flg_ovrdval>"
  Subsys VINP_SMUHSCFrP06Active_flg/1 -> Bus Creator/6  "VINP_SMUHSCFrP06Active_flg"
  Bus Selector2/1 -> Subsys VINP_BonnetOpen_flg/1  "<VHAL_BonnetOpenIn_flg>"
  Bus Selector8/1 -> Subsys VINP_BonnetOpen_flg/2  "<VSRV_BonnetOpenIn_flg_ovrdflg>"
  Bus Selector5/1 -> Subsys VINP_BonnetOpen_flg/3  "<VSRV_BonnetOpenIn_flg_ovrdval>"
  [MsgAlive_flgs] -> Subsys VINP_BonnetOpen_flg/4
  Subsys VINP_BonnetOpen_flg/1 -> Bus Creator/2  "VINP_BonnetOpenRaw_flg"
  Subsys VINP_BonnetOpen_flg/2 -> Bus Creator/3  "VINP_BonnetOpenRawValid_flg"

== system inp/INP/INP_100MS/Message (100ms) SMU_HSC_FrP07 ==
  BHAL_IN_100ms : Inport
  BSRV_In_ovrdflgs : Inport  Port=2
  BSRV_In_ovrdvals : Inport  Port=3
  VINP_SMUMsgAlive_flg : Inport  Port=4
  Bus Creator : BusCreator  Inputs=2
  Bus Selector1 : BusSelector  OutputSignals=VSRV_SMUHSCFrP07Active_flg_ovrdval
  Bus Selector2 : BusSelector  OutputSignals=VSRV_SMUHSCFrP07Active_flg_ovrdflg
  Bus Selector3 : BusSelector  OutputSignals=VHAL_SteerLockEngagedIn_flg
  Bus Selector5 : BusSelector  OutputSignals=VSRV_SteerLockEngagedIn_flg_ovrdflg
  Bus Selector6 : BusSelector  OutputSignals=VSRV_SteerLockEngagedIn_flg_ovrdval
  Subsys VINP_SMUHSCFrP07Active_flg : inp_lib/override  SystemSampleTime=-1  cal_ovrdflg=KINP_SMUHSCFrP07Active_ovrdflg  cal_ovrdval=KINP_SMUHSCFrP07Active_flg_ovrdval
  Subsys VINP_SteerLockEngaged_flg : inp_lib/msgactv_ovrd  SystemSampleTime=-1  cal_ovrdflg=KINP_SteerLockEngaged_flg_ovrdflg  cal_ovrdval=KINP_SteerLockEngaged_flg_ovrdval  default=KINP_SteerLockEngagedDefault_flg
  Terminator : Terminator
  BINP_SMU_HSC_FrP07 : Outport
  wires:
  [BSRV_In_ovrdvals] -> Bus Selector1/1
  [BSRV_In_ovrdflgs] -> Bus Selector2/1
  [VINP_SMUMsgAlive_flg] -> [MsgAlive_flgs], Subsys VINP_SMUHSCFrP07Active_flg/1
  BHAL_IN_100ms/1 -> Bus Selector3/1
  [BSRV_In_ovrdflgs] -> Bus Selector5/1
  [BSRV_In_ovrdvals] -> Bus Selector6/1
  VINP_SMUMsgAlive_flg/1 -> [VINP_SMUMsgAlive_flg]
  BSRV_In_ovrdflgs/1 -> [BSRV_In_ovrdflgs]
  BSRV_In_ovrdvals/1 -> [BSRV_In_ovrdvals]
  Bus Creator/1 -> BINP_SMU_HSC_FrP07/1  "BINP_SMU_HSC_FrP07"
  Bus Selector2/1 -> Subsys VINP_SMUHSCFrP07Active_flg/2  "<VSRV_SMUHSCFrP07Active_flg_ovrdflg>"
  Bus Selector1/1 -> Subsys VINP_SMUHSCFrP07Active_flg/3  "<VSRV_SMUHSCFrP07Active_flg_ovrdval>"
  Subsys VINP_SMUHSCFrP07Active_flg/1 -> Bus Creator/2  "VINP_SMUHSCFrP07Active_flg"
  Bus Selector3/1 -> Subsys VINP_SteerLockEngaged_flg/1  "<VHAL_SteerLockEngagedIn_flg>"
  Bus Selector5/1 -> Subsys VINP_SteerLockEngaged_flg/2  "<VSRV_SteerLockEngagedIn_flg_ovrdflg>"
  Bus Selector6/1 -> Subsys VINP_SteerLockEngaged_flg/3  "<VSRV_SteerLockEngagedIn_flg_ovrdval>"
  [MsgAlive_flgs] -> Subsys VINP_SteerLockEngaged_flg/4
  Subsys VINP_SteerLockEngaged_flg/1 -> Bus Creator/1  "VINP_SteerLockEngaged_flg"
  Subsys VINP_SteerLockEngaged_flg/2 -> Terminator/1

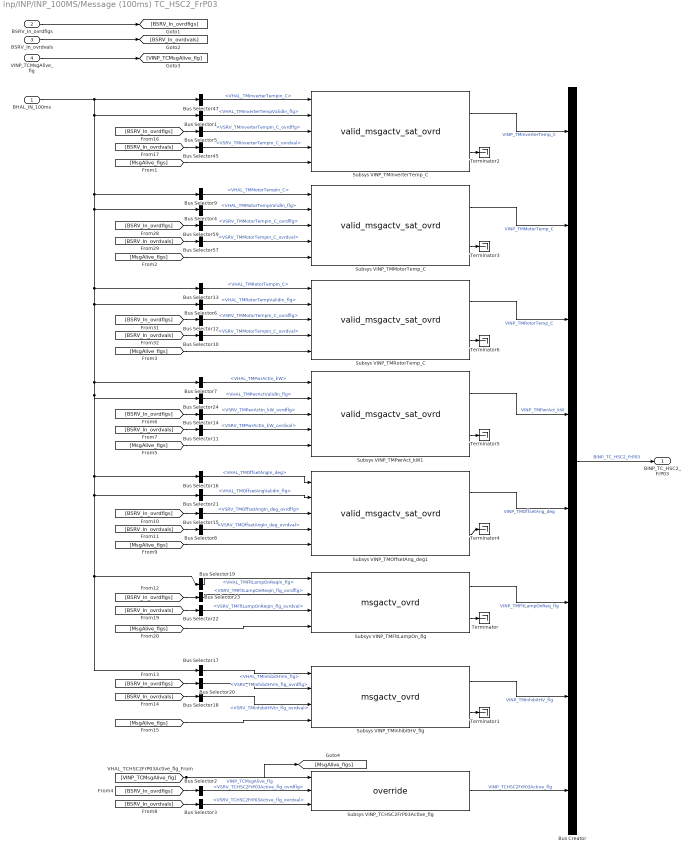
== system inp/INP/INP_100MS/Message (100ms) TC_HSC2_FrP03 ==
  BHAL_IN_100ms : Inport
  BSRV_In_ovrdflgs : Inport  Port=2
  BSRV_In_ovrdvals : Inport  Port=3
  VINP_TCMsgAlive_flg : Inport  Port=4
  Bus Creator : BusCreator  Inputs=8
  Bus Selector1 : BusSelector  OutputSignals=VHAL_TMInverterTempValidIn_flg
  Bus Selector10 : BusSelector  OutputSignals=VSRV_TMMotorTempIn_C_ovrdval
  Bus Selector11 : BusSelector  OutputSignals=VSRV_TMPwrActIn_kW_ovrdval
  Bus Selector12 : BusSelector  OutputSignals=VSRV_TMMotorTempIn_C_ovrdflg
  Bus Selector13 : BusSelector  OutputSignals=VHAL_TMRotorTempIn_C
  Bus Selector14 : BusSelector  OutputSignals=VSRV_TMPwrActIn_kW_ovrdflg
  Bus Selector15 : BusSelector  OutputSignals=VSRV_TMOffsetAngIn_deg_ovrdflg
  Bus Selector16 : BusSelector  OutputSignals=VHAL_TMOffsetAngIn_deg
  Bus Selector17 : BusSelector  OutputSignals=VHAL_TMInhibitHVIn_flg
  Bus Selector18 : BusSelector  OutputSignals=VSRV_TMInhibitHVIn_flg_ovrdval
  Bus Selector19 : BusSelector  OutputSignals=VHAL_TMFltLampOnReqIn_flg
  Bus Selector2 : BusSelector  OutputSignals=VSRV_TCHSC2FrP03Active_flg_ovrdflg
  Bus Selector20 : BusSelector  OutputSignals=VSRV_TMInhibitHVIn_flg_ovrdflg
  Bus Selector21 : BusSelector  OutputSignals=VHAL_TMOffsetAngValidIn_flg
  Bus Selector22 : BusSelector  OutputSignals=VSRV_TMFltLampOnReqIn_flg_ovrdval
  Bus Selector23 : BusSelector  OutputSignals=VSRV_TMFltLampOnReqIn_flg_ovrdflg
  Bus Selector24 : BusSelector  OutputSignals=VHAL_TMPwrActValidIn_flg
  Bus Selector3 : BusSelector  OutputSignals=VSRV_TCHSC2FrP03Active_flg_ovrdval
  Bus Selector4 : BusSelector  OutputSignals=VHAL_TMMotorTempValidIn_flg
  Bus Selector45 : BusSelector  OutputSignals=VSRV_TMInverterTempIn_C_ovrdval
  Bus Selector47 : BusSelector  OutputSignals=VHAL_TMInverterTempIn_C
  Bus Selector5 : BusSelector  OutputSignals=VSRV_TMInverterTempIn_C_ovrdflg
  Bus Selector57 : BusSelector  OutputSignals=VSRV_TMMotorTempIn_C_ovrdval
  Bus Selector59 : BusSelector  OutputSignals=VSRV_TMMotorTempIn_C_ovrdflg
  Bus Selector6 : BusSelector  OutputSignals=VHAL_TMRotorTempValidIn_flg
  Bus Selector7 : BusSelector  OutputSignals=VHAL_TMPwrActIn_kW
  Bus Selector8 : BusSelector  OutputSignals=VSRV_TMOffsetAngIn_deg_ovrdval
  Bus Selector9 : BusSelector  OutputSignals=VHAL_TMMotorTempIn_C
  Subsys VINP_TCHSC2FrP03Active_flg : inp_lib/override  SystemSampleTime=-1  cal_ovrdflg=KINP_TCHSC2FrP03Active_ovrdflg  cal_ovrdval=KINP_TCHSC2FrP03Active_flg_ovrdval
  Subsys VINP_TMFltLampOn_flg : inp_lib/msgactv_ovrd  SystemSampleTime=-1  cal_ovrdflg=KINP_TMFltLampOnReq_flg_ovrdflg  cal_ovrdval=KINP_TMFltLampOnReq_flg_ovrdval  default=KINP_TMFltLampOnReqDefault_flg
  Subsys VINP_TMInhibitHV_flg : inp_lib/msgactv_ovrd  SystemSampleTime=-1  cal_ovrdflg=KINP_TMInhibitHV_flg_ovrdflg  cal_ovrdval=KINP_TMInhibitHV_flg_ovrdval  default=KINP_TMInhibitHVDefault_flg
  Subsys VINP_TMInverterTemp_C : inp_lib/valid_msgactv_sat_ovrd  SystemSampleTime=-1  cal_ovrdflg=KINP_TMInverterTemp_C_ovrdflg  cal_ovrdval=KINP_TMInverterTemp_C_ovrdval  lim=KINP_ValidCheck_TMInverterTemp_lim  inc=KINP_ValidCheck_TMInverterTemp_inc  dec=KINP_ValidCheck_TMInverterTemp_dec  default=KINP_TMInverterTempDefault_C  hi=KINP_TMInverterTemp_C_Max  lo=KINP_TMInverterTemp_C_Min
  Subsys VINP_TMMotorTemp_C : inp_lib/valid_msgactv_sat_ovrd  SystemSampleTime=-1  cal_ovrdflg=KINP_TMMotorTemp_C_ovrdflg  cal_ovrdval=KINP_TMMotorTemp_C_ovrdval  lim=KINP_ValidCheck_TMMotorTemp_lim  inc=KINP_ValidCheck_TMMotorTemp_inc  dec=KINP_ValidCheck_TMMotorTemp_dec  default=KINP_TMMotorTempDefault_C  hi=KINP_TMMotorTemp_C_Max  lo=KINP_TMMotorTemp_C_Min
  Subsys VINP_TMOffsetAng_deg1 : inp_lib/valid_msgactv_sat_ovrd  SystemSampleTime=-1  cal_ovrdflg=KINP_TMOffsetAng_deg_ovrdflg  cal_ovrdval=KINP_TMOffsetAng_deg_ovrdval  lim=KINP_ValidCheck_TMOffsetAng_lim  inc=KINP_ValidCheck_TMOffsetAng_inc  dec=KINP_ValidCheck_TMOffsetAng_dec  default=KINP_TMOffsetAngDefault_deg  hi=KINP_TMOffsetAng_deg_Max  lo=KINP_TMOffsetAng_deg_Min
  Subsys VINP_TMPwrAct_kW1 : inp_lib/valid_msgactv_sat_ovrd  SystemSampleTime=-1  cal_ovrdflg=KINP_TMPwrAct_kW_ovrdflg  cal_ovrdval=KINP_TMPwrAct_kW_ovrdval  lim=KINP_ValidCheck_TMPwrAct_lim  inc=KINP_ValidCheck_TMPwrAct_inc  dec=KINP_ValidCheck_TMPwrAct_dec  default=KINP_TMPwrActDefault_kW  hi=KINP_TMPwrAct_kW_Max  lo=KINP_TMPwrAct_kW_Min
  Subsys VINP_TMRotorTemp_C : inp_lib/valid_msgactv_sat_ovrd  SystemSampleTime=-1  cal_ovrdflg=KINP_TMRotorTemp_C_ovrdflg  cal_ovrdval=KINP_TMRotorTemp_C_ovrdval  lim=KINP_ValidCheck_TMRotorTemp_lim  inc=KINP_ValidCheck_TMRotorTemp_inc  dec=KINP_ValidCheck_TMRotorTemp_dec  default=KINP_TMRotorTempDefault_C  hi=KINP_TMRotorTemp_C_Max  lo=KINP_TMRotorTemp_C_Min
  Terminator{,1..6} (7 alike) : Terminator
  BINP_TC_HSC2_FrP03 : Outport
  wires:
  Bus Selector24/1 -> Subsys VINP_TMPwrAct_kW1/2  "<VHAL_TMPwrActValidIn_flg>"
  Bus Selector21/1 -> Subsys VINP_TMOffsetAng_deg1/2  "<VHAL_TMOffsetAngValidIn_flg>"
  Bus Selector15/1 -> Subsys VINP_TMOffsetAng_deg1/3  "<VSRV_TMOffsetAngIn_deg_ovrdflg>"
  Bus Selector14/1 -> Subsys VINP_TMPwrAct_kW1/3  "<VSRV_TMPwrActIn_kW_ovrdflg>"
  [BSRV_In_ovrdvals] -> Bus Selector18/1
  [BSRV_In_ovrdflgs] -> Bus Selector20/1
  [BSRV_In_ovrdvals] -> Bus Selector22/1
  [BSRV_In_ovrdflgs] -> Bus Selector23/1
  [BSRV_In_ovrdvals] -> Bus Selector3/1
  [BSRV_In_ovrdflgs] -> Bus Selector2/1
  [VINP_TCMsgAlive_flg] -> [MsgAlive_flgs], Subsys VINP_TCHSC2FrP03Active_flg/1  "VINP_TCMsgAlive_flg"
  [BSRV_In_ovrdvals] -> Bus Selector57/1
  [BSRV_In_ovrdflgs] -> Bus Selector59/1
  [BSRV_In_ovrdvals] -> Bus Selector10/1
  [BSRV_In_ovrdflgs] -> Bus Selector12/1
  [BSRV_In_ovrdvals] -> Bus Selector45/1
  [BSRV_In_ovrdflgs] -> Bus Selector5/1
  BHAL_IN_100ms/1 -> Bus Selector1/1, Bus Selector13/1, Bus Selector6/1, Bus Selector24/1, Bus Selector21/1, Bus Selector17/1, Bus Selector19/1, Bus Selector16/1, Bus Selector7/1, Bus Selector4/1, Bus Selector9/1, Bus Selector47/1
  Bus Creator/1 -> BINP_TC_HSC2_FrP03/1  "BINP_TC_HSC2_FrP03"
  BSRV_In_ovrdvals/1 -> [BSRV_In_ovrdvals]
  BSRV_In_ovrdflgs/1 -> [BSRV_In_ovrdflgs]
  VINP_TCMsgAlive_flg/1 -> [VINP_TCMsgAlive_flg]
  [BSRV_In_ovrdvals] -> Bus Selector11/1
  [BSRV_In_ovrdflgs] -> Bus Selector14/1
  [BSRV_In_ovrdvals] -> Bus Selector8/1
  [BSRV_In_ovrdflgs] -> Bus Selector15/1
  Bus Selector2/1 -> Subsys VINP_TCHSC2FrP03Active_flg/2  "<VSRV_TCHSC2FrP03Active_flg_ovrdflg>"
  Bus Selector3/1 -> Subsys VINP_TCHSC2FrP03Active_flg/3  "<VSRV_TCHSC2FrP03Active_flg_ovrdval>"
  Subsys VINP_TCHSC2FrP03Active_flg/1 -> Bus Creator/8  "VINP_TCHSC2FrP03Active_flg"
  Bus Selector19/1 -> Subsys VINP_TMFltLampOn_flg/1  "<VHAL_TMFltLampOnReqIn_flg>"
  Bus Selector23/1 -> Subsys VINP_TMFltLampOn_flg/2  "<VSRV_TMFltLampOnReqIn_flg_ovrdflg>"
  Bus Selector22/1 -> Subsys VINP_TMFltLampOn_flg/3  "<VSRV_TMFltLampOnReqIn_flg_ovrdval>"
  [MsgAlive_flgs] -> Subsys VINP_TMFltLampOn_flg/4
  Subsys VINP_TMFltLampOn_flg/1 -> Bus Creator/6  "VINP_TMFltLampOnReq_flg"
  Subsys VINP_TMFltLampOn_flg/2 -> Terminator/1
  Bus Selector17/1 -> Subsys VINP_TMInhibitHV_flg/1  "<VHAL_TMInhibitHVIn_flg>"
  Bus Selector20/1 -> Subsys VINP_TMInhibitHV_flg/2  "<VSRV_TMInhibitHVIn_flg_ovrdflg>"
  Bus Selector18/1 -> Subsys VINP_TMInhibitHV_flg/3  "<VSRV_TMInhibitHVIn_flg_ovrdval>"
  [MsgAlive_flgs] -> Subsys VINP_TMInhibitHV_flg/4
  Subsys VINP_TMInhibitHV_flg/1 -> Bus Creator/7  "VINP_TMInhibitHV_flg"
  Subsys VINP_TMInhibitHV_flg/2 -> Terminator1/1
  Bus Selector47/1 -> Subsys VINP_TMInverterTemp_C/1  "<VHAL_TMInverterTempIn_C>"
  Bus Selector1/1 -> Subsys VINP_TMInverterTemp_C/2  "<VHAL_TMInverterTempValidIn_flg>"
  Bus Selector5/1 -> Subsys VINP_TMInverterTemp_C/3  "<VSRV_TMInverterTempIn_C_ovrdflg>"
  Bus Selector45/1 -> Subsys VINP_TMInverterTemp_C/4  "<VSRV_TMInverterTempIn_C_ovrdval>"
  [MsgAlive_flgs] -> Subsys VINP_TMInverterTemp_C/5
  Subsys VINP_TMInverterTemp_C/1 -> Bus Creator/1  "VINP_TMInverterTemp_C"
  Subsys VINP_TMInverterTemp_C/2 -> Terminator2/1
  Bus Selector9/1 -> Subsys VINP_TMMotorTemp_C/1  "<VHAL_TMMotorTempIn_C>"
  Bus Selector4/1 -> Subsys VINP_TMMotorTemp_C/2  "<VHAL_TMMotorTempValidIn_flg>"
  Bus Selector59/1 -> Subsys VINP_TMMotorTemp_C/3  "<VSRV_TMMotorTempIn_C_ovrdflg>"
  Bus Selector57/1 -> Subsys VINP_TMMotorTemp_C/4  "<VSRV_TMMotorTempIn_C_ovrdval>"
  [MsgAlive_flgs] -> Subsys VINP_TMMotorTemp_C/5
  Subsys VINP_TMMotorTemp_C/1 -> Bus Creator/2  "VINP_TMMotorTemp_C"
  Subsys VINP_TMMotorTemp_C/2 -> Terminator3/1
  Bus Selector16/1 -> Subsys VINP_TMOffsetAng_deg1/1  "<VHAL_TMOffsetAngIn_deg>"
  Bus Selector8/1 -> Subsys VINP_TMOffsetAng_deg1/4  "<VSRV_TMOffsetAngIn_deg_ovrdval>"
  [MsgAlive_flgs] -> Subsys VINP_TMOffsetAng_deg1/5
  Subsys VINP_TMOffsetAng_deg1/1 -> Bus Creator/5  "VINP_TMOffsetAng_deg"
  Subsys VINP_TMOffsetAng_deg1/2 -> Terminator4/1
  Bus Selector7/1 -> Subsys VINP_TMPwrAct_kW1/1  "<VHAL_TMPwrActIn_kW>"
  Bus Selector11/1 -> Subsys VINP_TMPwrAct_kW1/4  "<VSRV_TMPwrActIn_kW_ovrdval>"
  [MsgAlive_flgs] -> Subsys VINP_TMPwrAct_kW1/5
  Subsys VINP_TMPwrAct_kW1/1 -> Bus Creator/4  "VINP_TMPwrAct_kW"
  Subsys VINP_TMPwrAct_kW1/2 -> Terminator5/1
  Bus Selector13/1 -> Subsys VINP_TMRotorTemp_C/1  "<VHAL_TMRotorTempIn_C>"
  Bus Selector6/1 -> Subsys VINP_TMRotorTemp_C/2  "<VHAL_TMRotorTempValidIn_flg>"
  Bus Selector12/1 -> Subsys VINP_TMRotorTemp_C/3  "<VSRV_TMMotorTempIn_C_ovrdflg>"
  Bus Selector10/1 -> Subsys VINP_TMRotorTemp_C/4  "<VSRV_TMMotorTempIn_C_ovrdval>"
  [MsgAlive_flgs] -> Subsys VINP_TMRotorTemp_C/5
  Subsys VINP_TMRotorTemp_C/1 -> Bus Creator/3  "VINP_TMRotorTemp_C"
  Subsys VINP_TMRotorTemp_C/2 -> Terminator6/1

== system inp/INP/INP_100MS/Message (90ms) SMU_HSC_FrP00 ==
  BHAL_IN_100ms : Inport
  BSRV_In_ovrdflgs : Inport  Port=2
  BSRV_In_ovrdvals : Inport  Port=3
  VINP_SMUMsgAlive_flg : Inport  Port=4
  Bus Creator : BusCreator
  Bus Selector1 : BusSelector  OutputSignals=VHAL_FuelLevelValidIn_flg
  Bus Selector11 : BusSelector  OutputSignals=VSRV_FuelLevelIn_L_ovrdval
  Bus Selector12 : BusSelector  OutputSignals=VSRV_ATCACOnIn_flg_ovrdval
  Bus Selector14 : BusSelector  OutputSignals=VSRV_FuelLevelIn_L_ovrdflg
  Bus Selector16 : BusSelector  OutputSignals=VHAL_ATCACOnIn_flg
  Bus Selector18 : BusSelector  OutputSignals=VSRV_ATCACOnIn_flg_ovrdflg
  Bus Selector2 : BusSelector  OutputSignals=VSRV_SMUHSCFrP00Active_flg_ovrdflg
  Bus Selector3 : BusSelector  OutputSignals=VSRV_SMUHSCFrP00Active_flg_ovrdval
  Bus Selector7 : BusSelector  OutputSignals=VHAL_FuelLevelIn_L
  Subsys VINP_ATCACOn_flg : inp_lib/msgactv_ovrd  SystemSampleTime=-1  cal_ovrdflg=KINP_ATCACOn_flg_ovrdflg  cal_ovrdval=KINP_ATCACOn_flg_ovrdval  default=KINP_ATCACOnDefault_flg
  Subsys VINP_FuelLevel_L : inp_lib/valid_msgactv_sat_ovrd  SystemSampleTime=-1  cal_ovrdflg=KINP_FuelLevel_L_ovrdflg  cal_ovrdval=KINP_FuelLevel_L_ovrdval  lim=KINP_ValidCheck_FuelLevel_lim  inc=KINP_ValidCheck_FuelLevel_inc  dec=KINP_ValidCheck_FuelLevel_dec  default=KINP_FuelLevelDefault_L  hi=KINP_FuelLevel_L_Max  lo=KINP_FuelLevel_L_Min
  Subsys VINP_SMUHSCFrP00Active_flg : inp_lib/override  SystemSampleTime=-1  cal_ovrdflg=KINP_SMUHSCFrP00Active_ovrdflg  cal_ovrdval=KINP_SMUHSCFrP00Active_flg_ovrdval
  Terminator : Terminator
  BINP_SMU_HSC_FrP00 : Outport
  wires:
  [BSRV_In_ovrdvals] -> Bus Selector3/1
  [BSRV_In_ovrdflgs] -> Bus Selector2/1
  [VINP_SMUMsgAlive_flg] -> [MsgAlive_flgs], Subsys VINP_SMUHSCFrP00Active_flg/1
  [BSRV_In_ovrdvals] -> Bus Selector11/1
  [BSRV_In_ovrdflgs] -> Bus Selector14/1
  BHAL_IN_100ms/1 -> Bus Selector1/1, Bus Selector7/1, Bus Selector16/1
  [BSRV_In_ovrdvals] -> Bus Selector12/1
  [BSRV_In_ovrdflgs] -> Bus Selector18/1
  Bus Creator/1 -> BINP_SMU_HSC_FrP00/1  "BINP_SMU_HSC_FrP00"
  BSRV_In_ovrdvals/1 -> [BSRV_In_ovrdvals]
  BSRV_In_ovrdflgs/1 -> [BSRV_In_ovrdflgs]
  VINP_SMUMsgAlive_flg/1 -> [VINP_SMUMsgAlive_flg]
  Bus Selector16/1 -> Subsys VINP_ATCACOn_flg/1  "<VHAL_ATCACOnIn_flg>"
  Bus Selector18/1 -> Subsys VINP_ATCACOn_flg/2  "<VSRV_ATCACOnIn_flg_ovrdflg>"
  Bus Selector12/1 -> Subsys VINP_ATCACOn_flg/3  "<VSRV_ATCACOnIn_flg_ovrdval>"
  [MsgAlive_flgs] -> Subsys VINP_ATCACOn_flg/4
  Subsys VINP_ATCACOn_flg/1 -> Bus Creator/1  "VINP_ATCACOn_flg"
  Subsys VINP_ATCACOn_flg/2 -> Terminator/1
  Bus Selector7/1 -> Subsys VINP_FuelLevel_L/1  "<VHAL_FuelLevelIn_L>"
  Bus Selector1/1 -> Subsys VINP_FuelLevel_L/2  "<VHAL_FuelLevelValidIn_flg>"
  Bus Selector14/1 -> Subsys VINP_FuelLevel_L/3  "<VSRV_FuelLevelIn_L_ovrdflg>"
  Bus Selector11/1 -> Subsys VINP_FuelLevel_L/4  "<VSRV_FuelLevelIn_L_ovrdval>"
  [MsgAlive_flgs] -> Subsys VINP_FuelLevel_L/5
  Subsys VINP_FuelLevel_L/1 -> Bus Creator/2  "VINP_FuelLevel_L"
  Subsys VINP_FuelLevel_L/2 -> Bus Creator/3  "VINP_FuelLevelValid_flg"
  Bus Selector2/1 -> Subsys VINP_SMUHSCFrP00Active_flg/2  "<VSRV_SMUHSCFrP00Active_flg_ovrdflg>"
  Bus Selector3/1 -> Subsys VINP_SMUHSCFrP00Active_flg/3  "<VSRV_SMUHSCFrP00Active_flg_ovrdval>"
  Subsys VINP_SMUHSCFrP00Active_flg/1 -> Bus Creator/4  "VINP_SMUHSCFrP00Active_flg"
